simulink model "ex2_4"  (R2021a)
settings: Solver=VariableStepAuto  StartTime=0.0  StopTime=100  RelTol=1e-3
undefined symbols (not defined in the file or in its folder): b, D, I, invI, invM, k, L, mg, w
libraries: vrlib x1
settings Model: Creator=filippo  LastModifiedBy=filippo

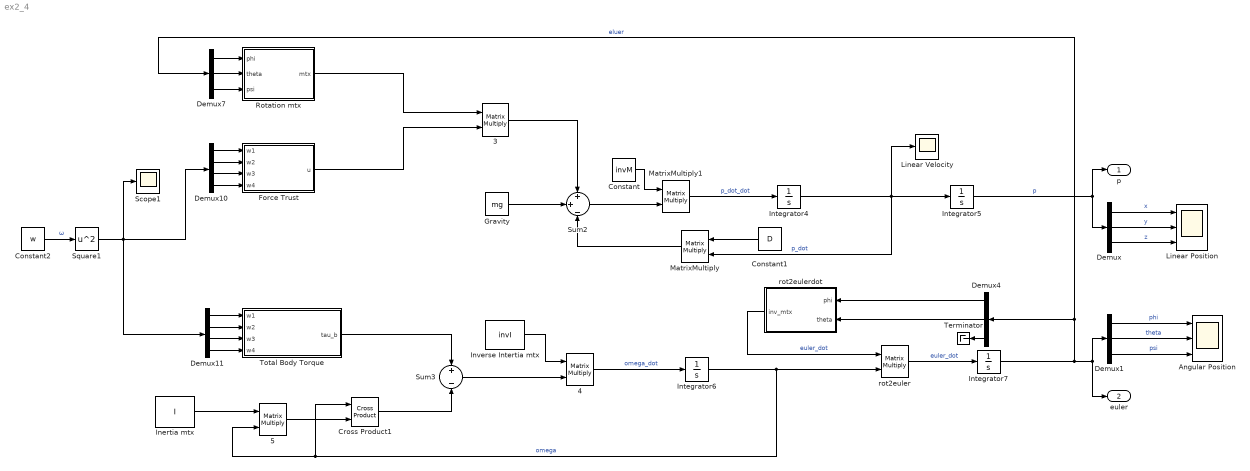
== system ex2_4 ==
  " 3" : Product  Multiplication=Matrix(*)
  " 4" : Product  Multiplication=Matrix(*)
  " 5" : Product  Multiplication=Matrix(*)
  Angular Position : Scope  NumInputPorts=3
  Constant : Constant  Value=invM
  Constant1 : Constant  Value=D
  Constant2 : Constant  Value=w
  Cross Product1 : vrlib/Utilities/Cross Product
  Demux{,1,4,7} (4 alike) : Demux  Outputs=3
  Demux10 : Demux
  Demux11 : Demux
  Force Trust : MATLAB Function  TreatAsAtomicUnit=on
  Gravity : Constant  Value=mg  VectorParams1D=off
  Inertia mtx : Constant  Value=I  VectorParams1D=off
  Integrator{4..7} (4 alike) : Integrator
  Inverse Intertia mtx : Constant  Value=invI
  Linear Position : Scope  NumInputPorts=3
  Linear Velocity : Scope
  MatrixMultiply : Product  Multiplication=Matrix(*)
  MatrixMultiply1 : Product  Multiplication=Matrix(*)
  Rotation mtx : MATLAB Function  TreatAsAtomicUnit=on
  Scope1 : Scope
  Square1 : Math  Operator=square  SaturateOnIntegerOverflow=on
  Sum2 : Sum  Inputs=+|+|-
  Sum3 : Sum  Inputs=+|-
  Terminator : Terminator
  Total Body Torque : MATLAB Function  TreatAsAtomicUnit=on
  rot2euler : Product  Multiplication=Matrix(*)
  rot2eulerdot : MATLAB Function  TreatAsAtomicUnit=on
  p : Outport
  euler : Outport  Port=2
  wires:
  Demux10/1 -> Force Trust/1(w1)
  " 5"/1 -> Cross Product1/2
  Demux10/4 -> Force Trust/4(w4)
  Demux10/2 -> Force Trust/2(w2)
  Demux11/2 -> Total Body Torque/2(w2)
  Inverse Intertia mtx/1 -> " 4"/1
  Force Trust/1(u) -> " 3"/2
  MatrixMultiply/1 -> Sum2/3
  Demux4/1 -> rot2eulerdot/1(phi)
  Demux7/1 -> Rotation mtx/1(phi)
  Cross Product1/1 -> Sum3/2
  Integrator5/1 -> Demux/1, p/1  "p"
  Total Body Torque/1(tau_b) -> Sum3/1
  Sum3/1 -> " 4"/2
  Demux11/1 -> Total Body Torque/1(w1)
  Inertia mtx/1 -> " 5"/1
  Integrator4/1 -> Linear Velocity/1, MatrixMultiply/2, Integrator5/1  "p_dot"
  Demux11/3 -> Total Body Torque/3(w3)
  MatrixMultiply1/1 -> Integrator4/1  "p_dot_dot"
  Demux4/2 -> rot2eulerdot/2(theta)
  Demux10/3 -> Force Trust/3(w3)
  Rotation mtx/1(mtx) -> " 3"/1
  Demux7/2 -> Rotation mtx/2(theta)
  Integrator6/1 -> rot2euler/2, Cross Product1/1, " 5"/2  "omega"
  " 4"/1 -> Integrator6/1  "omega_dot"
  Constant1/1 -> MatrixMultiply/1
  Demux7/3 -> Rotation mtx/3(psi)
  Demux11/4 -> Total Body Torque/4(w4)
  Gravity/1 -> Sum2/2
  Sum2/1 -> MatrixMultiply1/2
  " 3"/1 -> Sum2/1
  Constant2/1 -> Square1/1  "ω"
  Demux/2 -> Linear Position/2  "y"
  Demux/1 -> Linear Position/1  "x"
  Demux/3 -> Linear Position/3  "z"
  Demux1/3 -> Angular Position/3  "psi"
  Demux1/1 -> Angular Position/1  "phi"
  Demux1/2 -> Angular Position/2  "theta"
  Integrator7/1 -> Demux7/1, Demux4/1, euler/1, Demux1/1  "eluer"
  Square1/1 -> Demux10/1, Demux11/1, Scope1/1
  Constant/1 -> MatrixMultiply1/1
  Demux4/3 -> Terminator/1
  rot2eulerdot/1(inv_mtx) -> rot2euler/1  "euler_dot"
  rot2euler/1 -> Integrator7/1  "euler_dot"

== matlab function ex2_4/Force Trust ==
  data: w1 input; u output [..2]; w2 input; w3 input; w4 input; k parameter
function u = F_b(w1,w2,w3,w4,k)
u = k*[0; 0; w1+w2+w3+w4];
end

== matlab function ex2_4/Rotation mtx ==
  data: phi input; mtx output; theta input; psi input
function mtx = ROTATION(phi, theta, psi)
% Rot matrix Body-fixed frame wrt Inertial frame
mtx = Rz(psi) * Ry(theta) * Rx(phi);
end

== matlab function ex2_4/Total Body Torque ==
  data: w1 input; tau_b output; w2 input; w3 input; w4 input; L parameter; k parameter; b parameter
function tau_b= TotalBodyTorque(w1, w2, w3, w4, L, k, b)
tau_b = [L*k*(w1-w3); L*k*(w2-w4); b*(w1-w2+w3-w4)];
end

== matlab function ex2_4/rot2eulerdot ==
  data: phi input; inv_mtx output; theta input
function inv_mtx = rot2euler(phi, theta)
R = [1 0 -sin(theta); 
     0 cos(phi) cos(theta)*sin(phi);
     0 -sin(phi) cos(theta)*cos(phi)];
inv_mtx = inv(R);
end
